simulink model "controlofanonholonomicmobile"  (R2018b)
settings: Solver=FixedStepAuto  StartTime=0.0  StopTime=12  FixedStep=0.0012  RelTol=1e-3
settings Model: Creator=User  LastModifiedBy=User

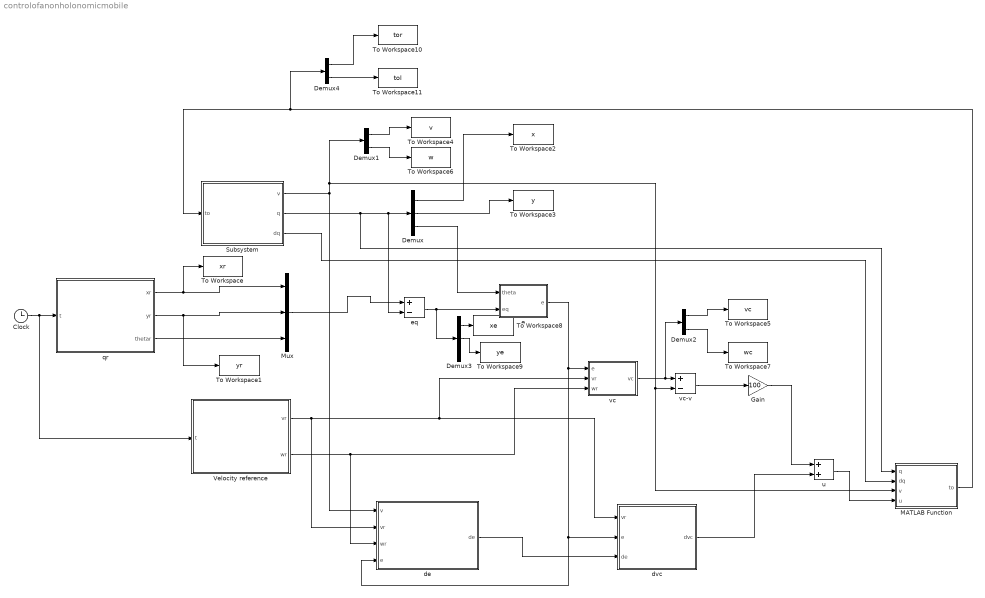
== system controlofanonholonomicmobile ==
  Clock : Clock
  Demux : Demux  Outputs=3
  Demux1 : Demux  Outputs=2
  Demux2 : Demux  Outputs=2
  Demux3 : Demux  Outputs=3
  Demux4 : Demux  Outputs=2
  Gain : Gain  Gain=100
  MATLAB Function : MATLAB Function  TreatAsAtomicUnit=on
  Mux : Mux  Inputs=3
  Subsystem : Subsystem
  To Workspace : ToWorkspace  VariableName=xr  SampleTime=-1
  To Workspace1 : ToWorkspace  VariableName=yr  SampleTime=-1
  To Workspace10 : ToWorkspace  VariableName=tor  SampleTime=-1
  To Workspace11 : ToWorkspace  VariableName=tol  SampleTime=-1
  To Workspace2 : ToWorkspace  VariableName=x  SampleTime=-1
  To Workspace3 : ToWorkspace  VariableName=y  SampleTime=-1
  To Workspace4 : ToWorkspace  VariableName=v  SampleTime=-1
  To Workspace5 : ToWorkspace  VariableName=vc  SampleTime=-1
  To Workspace6 : ToWorkspace  VariableName=w  SampleTime=-1
  To Workspace7 : ToWorkspace  VariableName=wc  SampleTime=-1
  To Workspace8 : ToWorkspace  VariableName=xe  SampleTime=-1
  To Workspace9 : ToWorkspace  VariableName=ye  SampleTime=-1
  Velocity reference : MATLAB Function  TreatAsAtomicUnit=on
  de : MATLAB Function  TreatAsAtomicUnit=on
  dvc : MATLAB Function  TreatAsAtomicUnit=on
  e : MATLAB Function  TreatAsAtomicUnit=on
  eq : Sum  Inputs=+-
  qr : MATLAB Function  TreatAsAtomicUnit=on
  u : Sum
  vc : MATLAB Function  TreatAsAtomicUnit=on
  vc-v : Sum  Inputs=+-
  wires:
  Clock/1 -> Velocity reference/1(t), qr/1(t)
  qr/1(xr) -> To Workspace/1, Mux/1
  qr/2(yr) -> To Workspace1/1, Mux/2
  qr/3(thetar) -> Mux/3
  Mux/1 -> eq/1
  Subsystem/2(q) -> MATLAB Function/1(q), Demux/1, eq/2
  eq/1 -> Demux3/1, e/2(eq)
  Demux/3 -> e/1(theta)
  e/1(e) -> dvc/2(e), de/4(e), vc/1(e)
  Velocity reference/1(vr) -> de/2(vr), dvc/1(vr), vc/2(vr)
  Velocity reference/2(wr) -> de/3(wr), vc/3(wr)
  vc/1(vc) -> Demux2/1, vc-v/1
  Subsystem/1(v) -> Demux1/1, MATLAB Function/3(v), vc-v/2, de/1(v)
  de/1(de) -> dvc/3(de)
  vc-v/1 -> Gain/1
  dvc/1(dvc) -> u/2
  Gain/1 -> u/1
  u/1 -> MATLAB Function/4(u)
  Subsystem/3(dq) -> MATLAB Function/2(dq)
  MATLAB Function/1(to) -> Demux4/1, Subsystem/1(to)
  Demux/1 -> To Workspace2/1
  Demux/2 -> To Workspace3/1
  Demux1/1 -> To Workspace4/1
  Demux2/1 -> To Workspace5/1
  Demux1/2 -> To Workspace6/1
  Demux2/2 -> To Workspace7/1
  Demux3/1 -> To Workspace8/1
  Demux3/2 -> To Workspace9/1
  Demux4/1 -> To Workspace10/1
  Demux4/2 -> To Workspace11/1

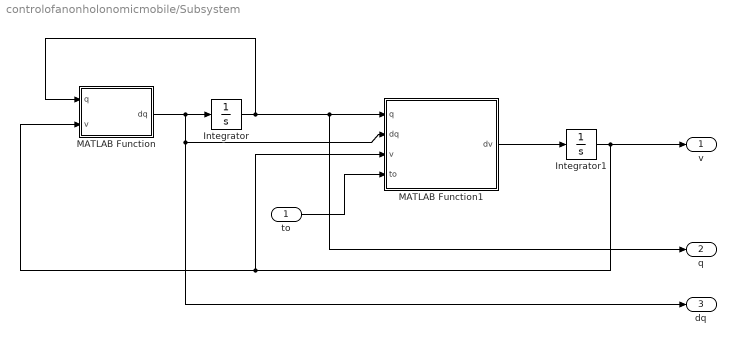
== system controlofanonholonomicmobile/Subsystem ==
  to : Inport
  Integrator : Integrator  InitialCondition=[1.15;0.85;0]
  Integrator1 : Integrator  InitialCondition=[0;0]
  MATLAB Function : MATLAB Function  TreatAsAtomicUnit=on
  MATLAB Function1 : MATLAB Function  TreatAsAtomicUnit=on
  v : Outport
  q : Outport  Port=2
  dq : Outport  Port=3
  wires:
  MATLAB Function/1(dq) -> dq/1, MATLAB Function1/2(dq), Integrator/1
  Integrator/1 -> q/1, MATLAB Function1/1(q), MATLAB Function/1(q)
  MATLAB Function1/1(dv) -> Integrator1/1
  Integrator1/1 -> v/1, MATLAB Function/2(v), MATLAB Function1/3(v)
  to/1 -> MATLAB Function1/4(to)

== matlab function controlofanonholonomicmobile/Subsystem/MATLAB Function1 ==
  data: q input; dv output; dq input; v input; to input
function dv = fcn(q,dq,v,to)
S=[cos(q(3)) -0.25*sin(q(3));
    sin(q(3)) 0.25*cos(q(3));
    0 1];
dS=[-dq(3)*sin(q(3)) -0.25*dq(3)*cos(q(3));
    dq(3)*cos(q(3)) -0.25*dq(3)*sin(q(3));
    0 0];
M=[1 0 1*0.25*sin(q(3));
    0 1 -1*0.25*cos(q(3));
    1*0.25*sin(q(3)) -1*0.25*cos(q(3)) 0.0587];
V=[0 0 1*0.25*dq(3)*cos(q(3));
   0 0 1*0.25*dq(3)*sin(q(3));
   0 0 0];
B=1/0.1*[cos(q(3)) cos(q(3));sin(q(3)) sin(q(3));0.5 -0.5];
Mq=S'*M*S;
Cq=S'*(M*dS+V*S);
Bq=S'*B;
dv=Mq\(Bq*to-Cq*v);
end

== matlab function controlofanonholonomicmobile/Subsystem/MATLAB Function ==
  data: q input; dq output; v input
function dq = fcn(q,v)
S=[cos(q(3)) -0.25*sin(q(3));
    sin(q(3)) 0.25*cos(q(3));
    0 1];
dq=S*v;
end

== matlab function controlofanonholonomicmobile/qr ==
  data: t input; xr output; yr output; thetar output
function [xr,yr,thetar] = fcn(t)
if t<2*sqrt(5)
    xr=1+1/sqrt(5)*t;
    yr=1+0.5/sqrt(5)*t;
    thetar=atan(0.5);
else
    xr=1.66+3*sin(atan(0.5)+0.125*(t-2*sqrt(5)));
    yr=4.68-3*cos(atan(0.5)+0.125*(t-2*sqrt(5)));
    thetar=atan(0.5)+0.125*(t-2*sqrt(5));
end
end

== matlab function controlofanonholonomicmobile/e ==
  data: theta input; e output; eq input
function e = fcn(theta,eq)
e=[cos(theta) sin(theta) 0;-sin(theta) cos(theta) 0;0 0 1]*eq;
end

== matlab function controlofanonholonomicmobile/Velocity reference ==
  data: t input; vr output; wr output
function [vr,wr] = fcn(t)
if t<2*sqrt(5)
    vr=0.5;
    wr=0;
else
    vr=0.375;
    wr=0.125;
end
end

== matlab function controlofanonholonomicmobile/vc ==
  data: e input; vc output; vr input; wr input
function vc = fcn(e,vr,wr)
vc=[vr*cos(e(3))+100*e(1);
    wr+100*vr*e(2)+100*vr*sin(e(3))];
end

== matlab function controlofanonholonomicmobile/de ==
  data: v input; de output; vr input; wr input; e input
function de = fcn(v,vr,wr,e)
de=[v(2)*e(2)-v(1)+vr*cos(e(3));
    -v(2)*e(1)+vr*sin(e(3));
    wr-v(2)];
end

== matlab function controlofanonholonomicmobile/dvc ==
  data: vr input; dvc output; e input; de input
function dvc  = fcn(vr,e,de)
dvc=[100 0 -vr*sin(e(3));
    0 100*vr 100*vr*cos(e(3))]*de;
end

== matlab function controlofanonholonomicmobile/MATLAB Function ==
  data: q input; dq input; v input; u input; to output
function to = fcn(q,dq,v,u)
S=[cos(q(3)) -0.25*sin(q(3));
    sin(q(3)) 0.25*cos(q(3));
    0 1];
dS=[-dq(3)*sin(q(3)) -0.25*dq(3)*cos(q(3));
    dq(3)*cos(q(3)) -0.25*dq(3)*sin(q(3));
    0 0];
M=[1 0 1*0.25*sin(q(3));
    0 1 -1*0.25*cos(q(3));
    1*0.25*sin(q(3)) -1*0.25*cos(q(3)) 0.0587];
V=[0 0 1*0.25*dq(3)*cos(q(3));
   0 0 1*0.25*dq(3)*sin(q(3));
   0 0 0];
B=1/0.1*[cos(q(3)) cos(q(3));sin(q(3)) sin(q(3));0.5 -0.5];
Mq=S'*M*S;
Cq=S'*(M*dS+V*S);
Bq=S'*B;
to=Bq\(Mq*u+Cq*v);
end
